simulink model "mavsim_chap9"  (R2014a)
settings: Solver=ode45  StartTime=0.0  StopTime=99999  RelTol=1e-3
InitFcn:
  | param_chap9
undefined symbols (not defined in the file or in its folder): autopilot, drawUAV, estimate_states, forces_moments, gps, P, plotextramavstatevariables, plotmavstatevariables, sensors, true_states
libraries: simulink x6
settings Model: Creator=beard  LastModifiedBy=danst_000
settings DataIOCC: SignalLoggingSaveFormat=ModelDataLogs
settings OptimizationCC: ExpressionDepthLimit=2147483647  InitFltsAndDblsToZero=on
settings DebuggingCC: UnderspecifiedInitializationDetection=Classic  FcnCallInpInsideContextMsg=UseLocalSettings  StateNameClashWarn=warning
settings SFSimCC: SimParseCustomCode=off
settings GRTTargetCC: CombineOutputUpdateFcns=off  GRTInterface=on

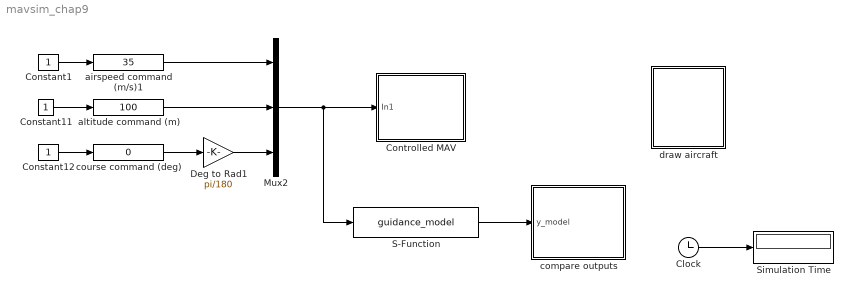
== system mavsim_chap9 ==
  Clock : Clock
  Constant1 : Constant
  Constant11 : Constant
  Constant12 : Constant
  Controlled MAV : Subsystem
      mask Display: image(imread('batcam.png'))
  Deg to Rad1 : Gain  Gain=pi/180
  Mux2 : Mux  Inputs=3
  S-Function : S-Function  FunctionName=guidance_model  Parameters=P  EnableBusSupport=off
  Simulation Time : Display
  airspeed command (m/s)1 : simulink/Math Operations/Slider Gain  low=30  gain=35  high=40
  altitude command (m) : simulink/Math Operations/Slider Gain  low=0  gain=100  high=120
  compare outputs : Subsystem
  course command (deg) : simulink/Math Operations/Slider Gain  low=-180  gain=0  high=180
  draw aircraft : Subsystem
      mask Display: image(imread('tv.jpg'))
  wires:
  Clock/1 -> Simulation Time/1
  Constant1/1 -> airspeed command (m/s)1/1
  Constant11/1 -> altitude command (m)/1
  Constant12/1 -> course command (deg)/1
  course command (deg)/1 -> Deg to Rad1/1
  altitude command (m)/1 -> Mux2/2
  airspeed command (m/s)1/1 -> Mux2/1
  Mux2/1 -> S-Function/1, Controlled MAV/1(In1)
  Deg to Rad1/1 -> Mux2/3
  S-Function/1 -> compare outputs/1(y_model)

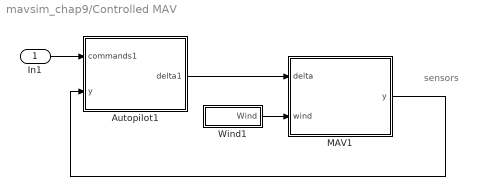
== system mavsim_chap9/Controlled MAV ==
  note: sensors
  In1 : Inport
  Autopilot1 : Subsystem
      mask Display: image(imread('kestrel.jpg'))
  MAV1 : Subsystem
      mask Display: image(imread('batcam.png'))
  Wind1 : Subsystem
  wires:
  In1/1 -> Autopilot1/1(commands1)
  Wind1/1(Wind) -> MAV1/2(wind)
  Autopilot1/1(delta1) -> MAV1/1(delta)
  MAV1/1(y) -> Autopilot1/2(y)

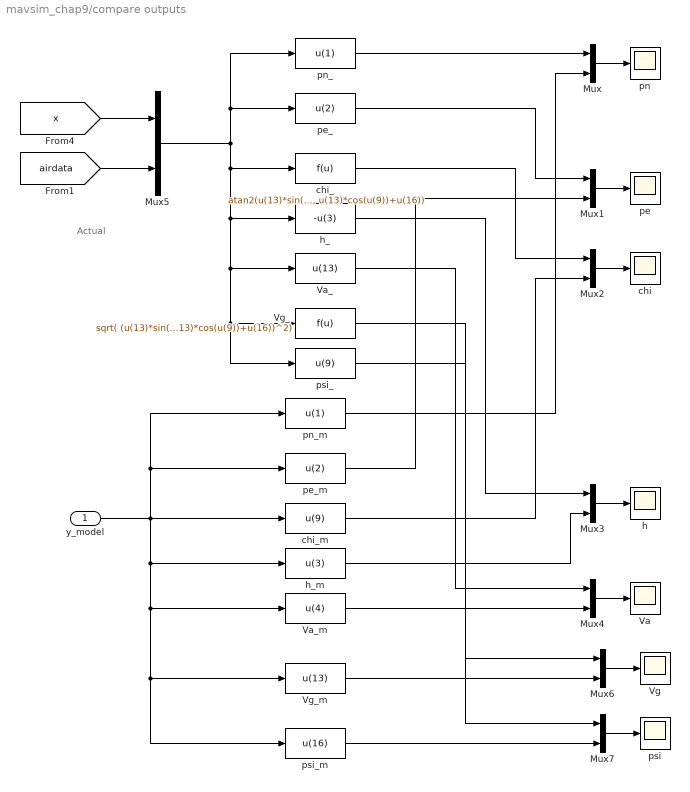
== system mavsim_chap9/compare outputs ==
  note: Actual
  y_model : Inport
  Mux{,1..7} (8 alike) : Mux  Inputs=2
  Va : Scope
      settings: TimeRange=40  YMin=25  YMax=72.5  SaveName=ScopeData4
  Va_ : Fcn  Expr=u(13)
  Va_m : Fcn  Expr=u(4)
  Vg : Scope
      settings: TimeRange=40  YMin=0  YMax=17  SaveName=ScopeData5
  Vg_ : Fcn  Expr=sqrt( (u(13)*sin(u(9))+u(17))^2+(u(13)*cos(u(9))+u(16))^2)
  Vg_m : Fcn  Expr=u(13)
  chi : Scope
      settings: TimeRange=40  YMin=-0.5  YMax=0.75  SaveName=ScopeData2
  chi_ : Fcn  Expr=atan2(u(13)*sin(u(9))+u(17), u(13)*cos(u(9))+u(16))
  chi_m : Fcn  Expr=u(9)
  h : Scope
      settings: TimeRange=115.3997603833866  YMin=-0  YMax=130  SaveName=ScopeData3
  h_ : Fcn  Expr=-u(3)
  h_m : Fcn  Expr=u(3)
  pe : Scope
      settings: TimeRange=40  YMin=-50  YMax=60
  pe_ : Fcn  Expr=u(2)
  pe_m : Fcn  Expr=u(2)
  pn : Scope
      settings: TimeRange=40  YMin=0  YMax=375
  pn_ : Fcn  Expr=u(1)
  pn_m : Fcn  Expr=u(1)
  psi : Scope
      settings: TimeRange=40  YMin=-0.025  YMax=0.225  SaveName=ScopeData6
  psi_ : Fcn  Expr=u(9)
  psi_m : Fcn  Expr=u(16)
  wires:
  pn_m/1 -> Mux/2
  chi_m/1 -> Mux2/2
  h_m/1 -> Mux3/2
  pe_m/1 -> Mux1/2
  Mux4/1 -> Va/1
  Mux3/1 -> h/1
  Mux2/1 -> chi/1
  Mux1/1 -> pe/1
  Mux/1 -> pn/1
  y_model/1 -> pn_m/1, pe_m/1, chi_m/1, h_m/1, Va_m/1, Vg_m/1, psi_m/1
  [x] -> Mux5/1
  [airdata] -> Mux5/2
  Mux5/1 -> pn_/1, pe_/1, h_/1, Va_/1, Vg_/1, psi_/1, chi_/1
  pn_/1 -> Mux/1
  pe_/1 -> Mux1/1
  Va_/1 -> Mux4/1
  h_/1 -> Mux3/1
  chi_/1 -> Mux2/1
  Vg_m/1 -> Mux6/2
  Mux6/1 -> Vg/1
  Vg_/1 -> Mux6/1
  psi_m/1 -> Mux7/2
  Mux7/1 -> psi/1
  psi_/1 -> Mux7/1
  Va_m/1 -> Mux4/2

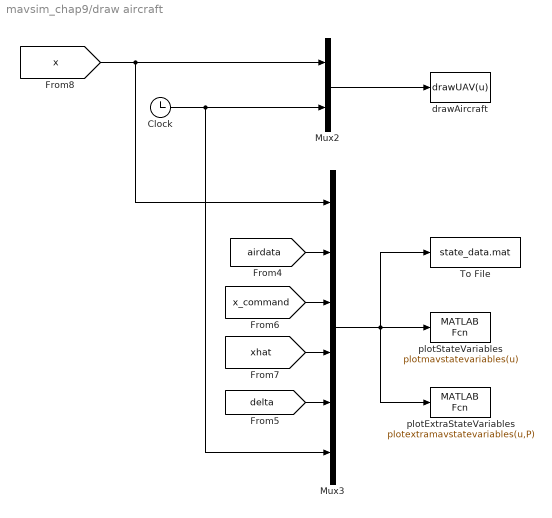
== system mavsim_chap9/draw aircraft ==
  Clock : Clock
  Mux2 : Mux  Inputs=2
  Mux3 : Mux  Inputs=6
  To File : ToFile  Filename=state_data.mat
  drawAircraft : MATLABFcn  MATLABFcn=drawUAV(u)  OutputDimensions=0  SampleTime=0.1
  plotExtraStateVariables : MATLABFcn  MATLABFcn=plotextramavstatevariables(u,P)  OutputDimensions=0  SampleTime=0.1
  plotStateVariables : MATLABFcn  MATLABFcn=plotmavstatevariables(u)  OutputDimensions=0  SampleTime=0.1
  wires:
  [airdata] -> Mux3/2
  [delta] -> Mux3/5
  [x_command] -> Mux3/3
  [xhat] -> Mux3/4
  Mux3/1 -> To File/1, plotExtraStateVariables/1, plotStateVariables/1
  Clock/1 -> Mux3/6, Mux2/2
  [x] -> Mux3/1, Mux2/1
  Mux2/1 -> drawAircraft/1

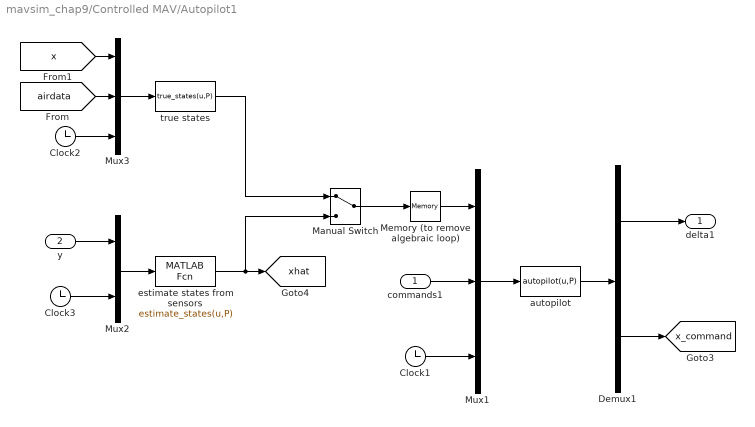
== system mavsim_chap9/Controlled MAV/Autopilot1 ==
  commands1 : Inport
  y : Inport  Port=2
  Clock1 : Clock
  Clock2 : Clock
  Clock3 : Clock
  Demux1 : Demux  Outputs=[4;12]
  Manual Switch : ManualSwitch
  Memory (to remove algebraic loop) : Memory
  Mux1 : Mux  Inputs=3
  Mux2 : Mux  Inputs=2
  Mux3 : Mux  Inputs=3
  autopilot : MATLABFcn  MATLABFcn=autopilot(u,P)  OutputDimensions=4+12  SampleTime=P.Ts
  estimate states from sensors : MATLABFcn  MATLABFcn=estimate_states(u,P)  OutputDimensions=19  SampleTime=P.Ts
  true states : MATLABFcn  MATLABFcn=true_states(u,P)  OutputDimensions=19  SampleTime=P.Ts
  delta1 : Outport
  tag scope: x_command=global, xhat=global
  wires:
  Mux1/1 -> autopilot/1
  autopilot/1 -> Demux1/1
  Demux1/1 -> delta1/1
  Demux1/2 -> [x_command]
  commands1/1 -> Mux1/2
  Mux2/1 -> estimate states from sensors/1
  y/1 -> Mux2/1
  Memory (to remove algebraic loop)/1 -> Mux1/1
  Manual Switch/1 -> Memory (to remove algebraic loop)/1
  true states/1 -> Manual Switch/1
  Mux3/1 -> true states/1
  [airdata] -> Mux3/2
  [x] -> Mux3/1
  Clock1/1 -> Mux1/3
  Clock2/1 -> Mux3/3
  Clock3/1 -> Mux2/2
  estimate states from sensors/1 -> Manual Switch/2, [xhat]

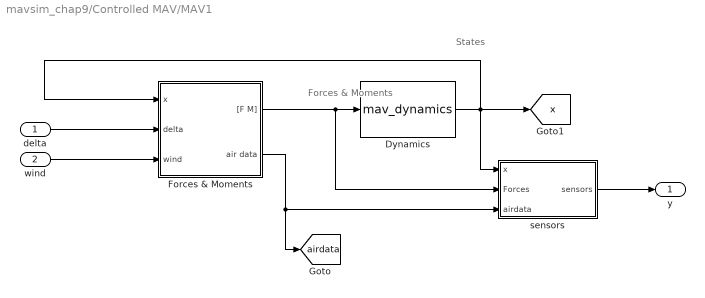
== system mavsim_chap9/Controlled MAV/MAV1 ==
  note: States
  note: Forces & Moments
  delta : Inport
  wind : Inport  Port=2
  Dynamics : S-Function  FunctionName=mav_dynamics  Parameters=P  EnableBusSupport=off
  Forces & Moments : Subsystem
  sensors : Subsystem
  y : Outport
  tag scope: airdata=global, x=global
  wires:
  wind/1 -> Forces & Moments/3(wind)
  delta/1 -> Forces & Moments/2(delta)
  Forces & Moments/2(air data) -> sensors/3(airdata), [airdata]
  Forces & Moments/1("[F M]") -> sensors/2(Forces), Dynamics/1
  Dynamics/1 -> [x], sensors/1(x), Forces & Moments/1(x)
  sensors/1(sensors) -> y/1

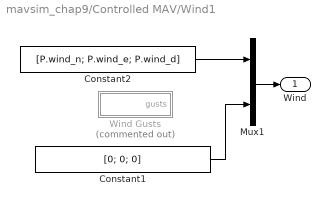
== system mavsim_chap9/Controlled MAV/Wind1 ==
  Constant1 : Constant  Value=[0; 0; 0]
  Constant2 : Constant  Value=[P.wind_n; P.wind_e; P.wind_d]
  Mux1 : Mux  Inputs=2
  Wind Gusts : Subsystem  Commented=on
  Wind : Outport
  wires:
  Constant1/1 -> Mux1/2
  Mux1/1 -> Wind/1
  Constant2/1 -> Mux1/1

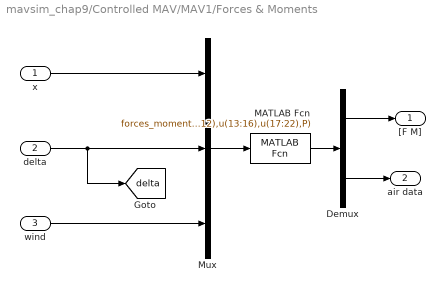
== system mavsim_chap9/Controlled MAV/MAV1/Forces & Moments ==
  x : Inport
  delta : Inport  Port=2
  wind : Inport  Port=3
  Demux : Demux  Outputs=[6;6]
  MATLAB Fcn : MATLABFcn  MATLABFcn=forces_moments(u(1:12),u(13:16),u(17:22),P)  OutputDimensions=12
  Mux : Mux  Inputs=3
  "[F M]" : Outport
  air data : Outport  Port=2
  tag scope: delta=global
  wires:
  Demux/2 -> air data/1
  Mux/1 -> MATLAB Fcn/1
  Demux/1 -> "[F M]"/1
  MATLAB Fcn/1 -> Demux/1
  wind/1 -> Mux/3
  delta/1 -> Mux/2, [delta]
  x/1 -> Mux/1

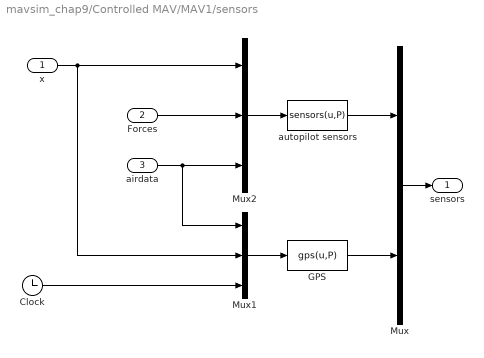
== system mavsim_chap9/Controlled MAV/MAV1/sensors ==
  x : Inport
  Forces : Inport  Port=2
  airdata : Inport  Port=3
  Clock : Clock
  GPS : MATLABFcn  MATLABFcn=gps(u,P)  OutputDimensions=5  SampleTime=P.Ts_gps
  Mux : Mux  Inputs=2
  Mux1 : Mux  Inputs=3
  Mux2 : Mux  Inputs=3
  autopilot sensors : MATLABFcn  MATLABFcn=sensors(u,P)  OutputDimensions=8  SampleTime=P.Ts
  sensors : Outport
  wires:
  x/1 -> Mux1/2, Mux2/1
  Mux/1 -> sensors/1
  airdata/1 -> Mux1/1, Mux2/3
  Forces/1 -> Mux2/2
  Mux2/1 -> autopilot sensors/1
  Clock/1 -> Mux1/3
  Mux1/1 -> GPS/1
  GPS/1 -> Mux/2
  autopilot sensors/1 -> Mux/1

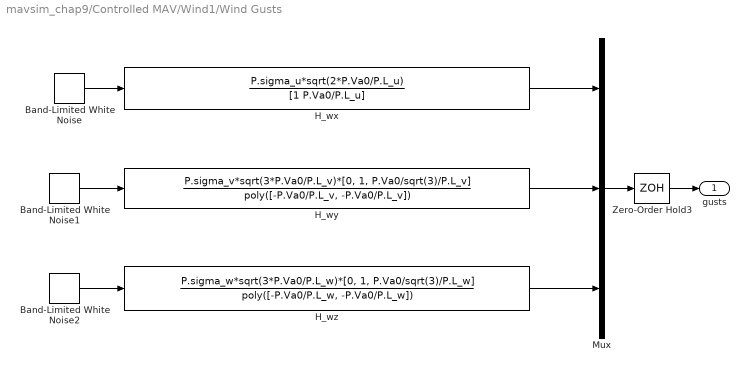
== system mavsim_chap9/Controlled MAV/Wind1/Wind Gusts ==
  Band-Limited White Noise : simulink/Sources/Band-Limited White Noise  Cov=[1]  Ts=P.Ts  seed=[23341]
  Band-Limited White Noise1 : simulink/Sources/Band-Limited White Noise  Cov=[1]  Ts=P.Ts  seed=[23341]
  Band-Limited White Noise2 : simulink/Sources/Band-Limited White Noise  Cov=[1]  Ts=P.Ts  seed=[23341]
  H_wx : TransferFcn  Numerator=P.sigma_u*sqrt(2*P.Va0/P.L_u)  Denominator=[1 P.Va0/P.L_u]
  H_wy : TransferFcn  Numerator=P.sigma_v*sqrt(3*P.Va0/P.L_v)*[0, 1, P.Va0/sqrt(3)/P.L_v]  Denominator=poly([-P.Va0/P.L_v, -P.Va0/P.L_v])
  H_wz : TransferFcn  Numerator=P.sigma_w*sqrt(3*P.Va0/P.L_w)*[0, 1, P.Va0/sqrt(3)/P.L_w]  Denominator=poly([-P.Va0/P.L_w, -P.Va0/P.L_w])
  Mux : Mux  Inputs=3
  Zero-Order Hold3 : ZeroOrderHold  SampleTime=P.Ts
  gusts : Outport
  wires:
  H_wx/1 -> Mux/1
  Band-Limited White Noise/1 -> H_wx/1
  H_wy/1 -> Mux/2
  Band-Limited White Noise1/1 -> H_wy/1
  H_wz/1 -> Mux/3
  Band-Limited White Noise2/1 -> H_wz/1
  Mux/1 -> Zero-Order Hold3/1
  Zero-Order Hold3/1 -> gusts/1
